simulink model "pid_ej1_simulink"  (Simulink 8.3)
settings: Solver=ode45  StartTime=0.0  StopTime=10  RelTol=1e-3
values from neighbouring files (symbols this model uses):
  Kd = 0.2*11    (= 2.2)    [pid_1.m]    (also in variables_pid_ej1.mat)
  Ki = 100    [pid_1.m]    (also in variables_pid_ej1.mat)
  Kp = 11 + 0.2*100    (= 31)    [pid_1.m]    (also in variables_pid_ej1.mat)
libraries: simulink x1
settings Model: Creator=IvanBurgos  LastModifiedBy=IvanBurgos
settings DataIOCC: SignalLoggingSaveFormat=Dataset
settings DebuggingCC: UnderspecifiedInitializationDetection=Simplified  StateNameClashWarn=none
settings GRTTargetCC: CombineOutputUpdateFcns=on  GRTInterface=off

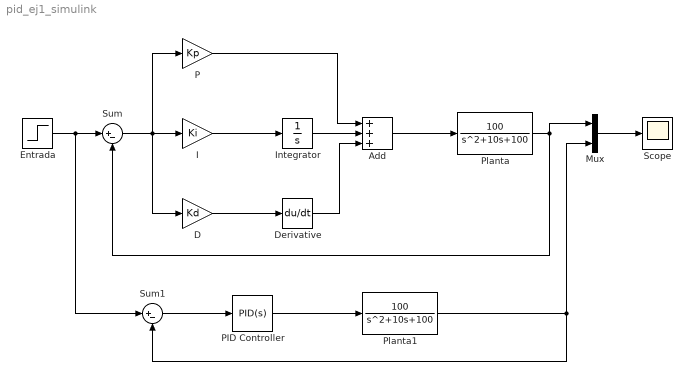
== system pid_ej1_simulink ==
  Add : Sum  Inputs=+++
  D : Gain  Gain=Kd
  Derivative : Derivative
  "Entrada " : Step  SampleTime=0
  I : Gain  Gain=Ki
  Integrator : Integrator
  Mux : Mux  Inputs=2
  P : Gain  Gain=Kp
  PID Controller : simulink/Continuous/PID Controller  Controller=PID  TimeDomain=Continuous-time  SampleTime=1  IntegratorMethod=Forward Euler  FilterMethod=Forward Euler  Form=Parallel  P=15.0492576879621  I=10.5832648320599  D=0.798705759113597  N=877.131255821739  InitialConditionSource=internal  InitialConditionForIntegrator=0  InitialConditionForFilter=0  ExternalReset=none  LimitOutput=off  UpperSaturationLimit=inf  LowerSaturationLimit=-inf  LinearizeAsGain=on  AntiWindupMode=none  Kb=1  TrackingMode=off  Kt=1  PParamMin=[]  PParamMax=[]  IParamMin=[]  IParamMax=[]  DParamMin=[]  DParamMax=[]  NParamMin=[]  NParamMax=[]  KbParamMin=[]  KbParamMax=[]  KtParamMin=[]  KtParamMax=[]  POutMin=[]  POutMax=[]  IOutMin=[]  IOutMax=[]  DOutMin=[]  DOutMax=[]  NOutMin=[]  NOutMax=[]  KbOutMin=[]  KbOutMax=[]  KtOutMin=[]  KtOutMax=[]  IntegratorOutMin=[]  IntegratorOutMax=[]  FilterOutMin=[]  FilterOutMax=[]  SumOutMin=[]  SumOutMax=[]  SumI1OutMin=[]  SumI1OutMax=[]  SumI2OutMin=[]  SumI2OutMax=[]  SumI3OutMin=[]  SumI3OutMax=[]  SumDOutMin=[]  SumDOutMax=[]  SaturationOutMin=[]  SaturationOutMax=[]  IntegratorContinuousStateAttributes=''  IntegratorStateMustResolveToSignalObject=off  IntegratorRTWStateStorageClass=Auto  FilterContinuousStateAttributes=''  FilterStateMustResolveToSignalObject=off  FilterRTWStateStorageClass=Auto
  Planta : TransferFcn  Numerator=[100]  Denominator=[1 10 100]
  Planta1 : TransferFcn  Numerator=[100]  Denominator=[1 10 100]
  Scope : Scope
  Sum : Sum  Inputs=|+-
  Sum1 : Sum  Inputs=|+-
  wires:
  Sum/1 -> D/1, I/1, P/1
  I/1 -> Integrator/1
  P/1 -> Add/1
  Integrator/1 -> Add/2
  Derivative/1 -> Add/3
  D/1 -> Derivative/1
  Add/1 -> Planta/1
  Planta/1 -> Sum/2, Mux/1
  "Entrada "/1 -> Sum1/1, Sum/1
  PID Controller/1 -> Planta1/1
  Planta1/1 -> Mux/2, Sum1/2
  Mux/1 -> Scope/1
  Sum1/1 -> PID Controller/1
